simulink model "BrakeActuatorSubplant"  (Simulink 8.5)
settings: Solver=ode45  StartTime=0.0  StopTime=20  RelTol=1e-3
settings Model: Creator=MrPiccolo  LastModifiedBy=MrPiccolo
settings DataIOCC: SignalLoggingSaveFormat=Dataset
settings OptimizationCC: ExpressionDepthLimit=128
settings DebuggingCC: UnderspecifiedInitializationDetection=Simplified  MergeDetectMultiDrivingBlocksExec=error  FcnCallInpInsideContextMsg=EnableAllAsError  StateNameClashWarn=none
settings GRTTargetCC: CombineOutputUpdateFcns=on  GRTInterface=off

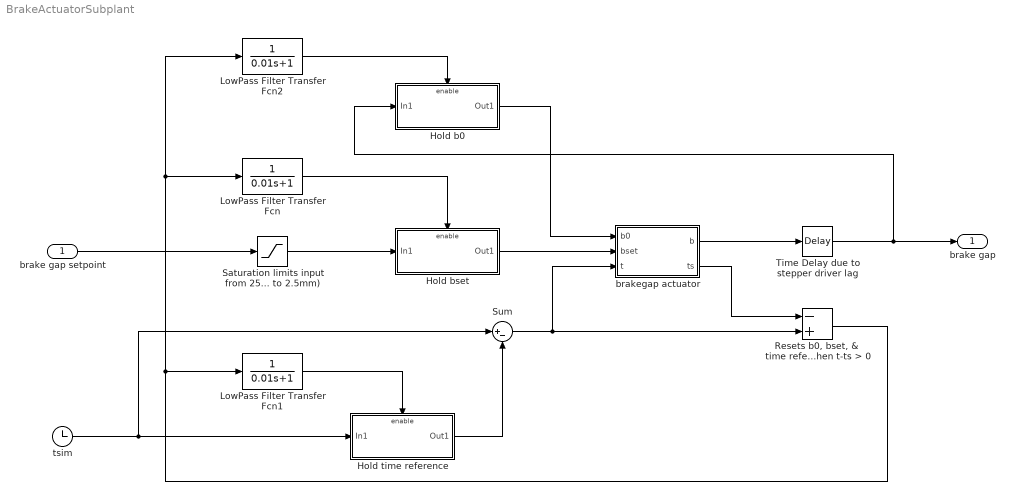
== system BrakeActuatorSubplant ==
  brake gap setpoint : Inport
  Hold b0 : Subsystem  TreatAsAtomicUnit=on
  Hold bset : Subsystem  TreatAsAtomicUnit=on
  Hold time reference : Subsystem  TreatAsAtomicUnit=on
  LowPass Filter Transfer Fcn : TransferFcn  Denominator=[0.01 1]
  LowPass Filter Transfer Fcn1 : TransferFcn  Denominator=[0.01 1]
  LowPass Filter Transfer Fcn2 : TransferFcn  Denominator=[0.01 1]
  "Resets b0, bset, &  time reference when t-ts > 0" : Sum  Inputs=-+
  Saturation limits input from 25mm to 2.5mm) : Saturate  UpperLimit=25  LowerLimit=2.5
  Sum : Sum  Inputs=|+-
  Time Delay due to stepper driver lag : TransportDelay  DelayTime=.05  InitialOutput=25
  brakegap actuator : MATLAB Function  TreatAsAtomicUnit=on
  tsim : Clock
  brake gap : Outport
  wires:
  brake gap setpoint/1 -> Saturation limits input from 25mm to 2.5mm)/1
  Saturation limits input from 25mm to 2.5mm)/1 -> Hold bset/1(In1)
  LowPass Filter Transfer Fcn/1 -> Hold bset/Enable
  Hold bset/1(Out1) -> brakegap actuator/2(bset)
  brakegap actuator/1(b) -> Time Delay due to stepper driver lag/1
  LowPass Filter Transfer Fcn2/1 -> Hold b0/Enable
  Hold b0/1(Out1) -> brakegap actuator/1(b0)
  "Resets b0, bset, &  time reference when t-ts > 0"/1 -> LowPass Filter Transfer Fcn2/1, LowPass Filter Transfer Fcn/1, LowPass Filter Transfer Fcn1/1
  Hold time reference/1(Out1) -> Sum/2
  tsim/1 -> Hold time reference/1(In1), Sum/1
  Time Delay due to stepper driver lag/1 -> brake gap/1, Hold b0/1(In1)
  brakegap actuator/2(ts) -> "Resets b0, bset, &  time reference when t-ts > 0"/1
  LowPass Filter Transfer Fcn1/1 -> Hold time reference/Enable
  Sum/1 -> "Resets b0, bset, &  time reference when t-ts > 0"/2, brakegap actuator/3(t)

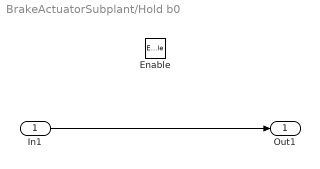
== system BrakeActuatorSubplant/Hold b0 ==
  In1 : Inport
  Enable : EnablePort
  Out1 : Outport
  wires:
  In1/1 -> Out1/1

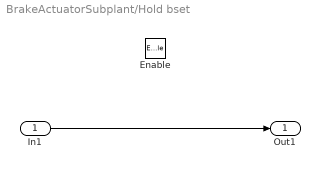
== system BrakeActuatorSubplant/Hold bset ==
  In1 : Inport
  Enable : EnablePort
  Out1 : Outport
  wires:
  In1/1 -> Out1/1

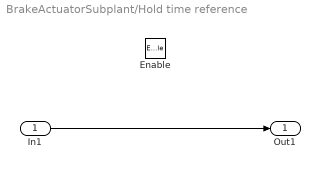
== system BrakeActuatorSubplant/Hold time reference ==
  In1 : Inport
  Enable : EnablePort
  Out1 : Outport
  wires:
  In1/1 -> Out1/1

== matlab function brakegap actuator ==
  data: b0 input double; b output double; bset input double; t input double; ts output double
function [b,ts] = fcn(b0,bset,t)
%#codegen

% Calculate settling time and read brakegap at time t
[b,ts] = brakeactuator(b0,bset,t);
